simulink model "nucleo_stm32g474_pid_v3_19_05"  (R2025b)
settings: Solver=FixedStepAuto  StartTime=0.0  StopTime=inf  FixedStep=1e-4  RelTol=1e-3  EnableMultiTasking=on
values from neighbouring files (symbols this model uses):
  Ts = single(1e-4)    [smc_mancal.m]
undefined symbols (not defined in the file or in its folder): alpha, dspblkCoreblockFVToolHelper, gcbh
libraries: stm32f4xxblockslib x10, simulink x1
settings Model: STM32="{\"AnalogInput\":[{\"ID\":\"untitled:286\"},{\"ID\":\"untitled:287\"},{\"ID\":\"untitled:288\"},{\"ID\":\"untitled:289\"},{\"ID\":\"nucleo_stm32g474_smc_v1_05_01:311\"},{\"ID\":\"nucleo_stm32g474_smc_v1_05_01:312\"},{\"ID\":\"nucleo_stm32g474_smc_v1_05_01:313\"},{\"ID\":\"nucleo_stm32g474_smc_v1_05_01:314\"},{\"ID\":\"nucleo_stm32g474_smc_v2_06_01:314\"},{\"ID\":\"nucleo_stm32g474_smc_v2_06_01:313\"},{\"ID\":\"nucleo_stm32g474_smc_v2_06_01:312\"},{\"ID\":\"nucleo_stm32g474_smc_v2_06_01:311\"},{\"ID\":\"nucleo_stm32g474_pid_v1_15_01:311\"},{\"ID\":\"nucleo_stm32g474_pid_v1_15_01:312\"},{\"ID\":\"nucleo_stm32g474_pid_v1_15_01:313\"},{\"ID\":\"nucleo_stm32g474_pid_v1_15_01:314\"},{\"ID\":\"nucleo_stm32g474_pid_v1_21_01:311\"},{\"ID\":\"nucleo_stm32g474_pid_v1_21_01:312\"},{\"ID\":\"nucleo_stm32g474_pid_v1_21_01:313\"},{\"ID\":\"nucleo_stm32g474_pid_v1_21_01:314\"},{\"ID\":\"nucleo_stm32g474_pid_v1_29_01:311\"},{\"ID\":\"nucleo_stm32g474_pid_v1_29_01:312\"},{\"ID\":\"nucleo_stm32g474_pid_v1_29_01:313\"},{\"ID\":\"nucleo_stm32g474_pid_v1_29_01:314\"},{\"ID\":\"nucleo_stm32g474_pid_v2_17_03:311\"},{\"ID\":\"nucleo_stm32g474_pid_v2_17_03:312\"},{\"ID\":\"nucleo_stm32g474_pid_v2_17_03:313\"},{\"ID\":\"nucleo_stm32g474_pid_v2_17_03:314\"},{\"ID\":\"nucleo_stm32g474_pid_v3_11_05:311\"},{\"ID\":\"nucleo_stm32g474_pid_v3_11_05:312\"},{\"ID\":\"nucleo_stm32g474_pid_v3_11_05:313\"},{\"ID\":\"nucleo_stm32g474_pid_v3_11_05:314\"},{\"ID\":\"nucleo_stm32g474_pid_v3_19_05:311\"},{\"ID\":\"nucleo_stm32g474_pid_v3_19_05:312\"},{\"ID\":\"nucleo_stm32g474_pid_v3_19_05:313\"},{\"ID\":\"nucleo_stm32g474_pid_v3_19_05:314\"}],\"PWMOutput\":[{\"ID\":\"untitled:236\"},{\"ID\":\"untitled:235\"},{\"ID\":\"untitled:234\"},{\"ID\":\"untitled:233\"},{\"ID\":\"nucleo_stm32g474_smc_v1_05_01:353\"},{\"ID\":\"nucleo_stm32g474_smc_v1_05_01:354\"},{\"ID\":\"nucleo_stm32g474_smc_v1_05_01:355\"},{\"ID\":\"nucleo_stm32g474_smc_v1_05_01:356\"},{\"ID\":\"nucleo_stm32g474_smc_v2_06_01:480\"},{\"ID\":\"nucleo_stm32g474_smc_v2_06_01:481\"},{\"ID\":\"nucleo_stm32g474_smc_v2_06_01:482\"},{\"ID\":\"nucleo_stm32g474_smc_v2_06_01:483\"},{\"ID\":\"nucleo_stm32g474_smc_v2_06_01:488\"},{\"ID\":\"nucleo_stm32g474_pid_v1_15_01:480\"},{\"ID\":\"nucleo_stm32g474_pid_v1_15_01:481\"},{\"ID\":\"nucleo_stm32g474_pid_v1_15_01:482\"},{\"ID\":\"nucleo_stm32g474_pid_v1_15_01:483\"},{\"ID\":\"nucleo_stm32g474_pid_v1_15_01:488\"},{\"ID\":\"nucleo_stm32g474_pid_v1_21_01:480\"},{\"ID\":\"nucleo_stm32g474_pid_v1_21_01:481\"},{\"ID\":\"nucleo_stm32g474_pid_v1_21_01:482\"},{\"ID\":\"nucleo_stm32g474_pid_v1_21_01:483\"},{\"ID\":\"nucleo_stm32g474_pid_v1_21_01:488\"},{\"ID\":\"nucleo_stm32g474_pid_v1_29_01:480\"},{\"ID\":\"nucleo_stm32g474_pid_v1_29_01:481\"},{\"ID\":\"nucleo_stm32g474_pid_v1_29_01:482\"},{\"ID\":\"nucleo_stm32g474_pid_v1_29_01:483\"},{\"ID\":\"nucleo_stm32g474_pid_v1_29_01:488\"},{\"ID\":\"nucleo_stm32g474_pid_v2_17_03:488\"},{\"ID\":\"nucleo_stm32g474_pid_v2_17_03:483\"},{\"ID\":\"nucleo_stm32g474_pid_v2_17_03:482\"},{\"ID\":\"nucleo_stm32g474_pid_v2_17_03:481\"},{\"ID\":\"nucleo_stm32g474_pid_v2_17_03:480\"},{\"ID\":\"nucleo_stm32g474_pid_v3_11_05:480\"},{\"ID\":\"nucleo_stm32g474_pid_v3_11_05:481\"},{\"ID\":\"nucleo_stm32g474_pid_v3_11_05:482\"},{\"ID\":\"nucleo_stm32g474_pid_v3_11_05:483\"},{\"ID\":\"nucleo_stm32g474_pid_v3_11_05:488\"},{\"ID\":\"nucleo_stm32g474_pid_v3_19_05:488\"},{\"ID\":\"nucleo_stm32g474_pid_v3_19_05:483\"},{\"ID\":\"nucleo_stm32g474_pid_v3_19_05:482\"},{\"ID\":\"nucleo_stm32g474_pid_v3_19_05:481\"},{\"ID\":\"nucleo_stm32g474_pid_v3_19_05:480\"}],\"DigitalPortWrite\":{\"ID\":\"nucleo_stm32g474_pid_v3_19_05:665\"}}"  SimulationMode=external  TunableVars=F,lambda,zeta  TunableVarsStorageClass=Auto,Auto,Auto  TunableVarsTypeQualifier=,,  Creator=thaty  LastModifiedBy=thaty
settings OptimizationCC: EnhancedBackFolding=on  PassReuseOutputArgsAs=Individual arguments  ZeroExternalMemoryAtStartup=off  ZeroInternalMemoryAtStartup=off  MaxStackSize=512  OptimizeBlockOrder=speed  DifferentSizesBufferReuse=on  OptimizationCustomize=off  EfficientTunableParamExpr=on
settings DebuggingCC: ParameterTunabilityLossMsg=error
settings HardwareCC: ProdBitPerPointer=32.0  ProdBitPerSizeT=32.0  ProdBitPerPtrDiffT=32.0  ProdLargestAtomicInteger=Long  ProdLargestAtomicFloat=Double  ProdWordSize=32.0  ProdLongLongMode=on  ProdHWDeviceType=ARM Compatible->ARM Cortex-M
settings SFSimCC: MATLABDynamicMemAlloc=off
settings RTWCC: SystemTargetFile=ert.tlc  HardwareBoard=STM32G4xx Based  TemplateMakefile=ert_default_tmf  Toolchain=GNU Tools for ARM Embedded Processors  BuildConfiguration=Faster Runs  Description=Embedded Coder
settings RTWCC: CustomInitializer=|
  | LL_OPAMP_Enable(OPAMP1);
  | LL_OPAMP_Enable(OPAMP2);
  | LL_OPAMP_Enable(OPAMP3);
  | LL_OPAMP_Enable(OPAMP6);
settings CodeAppCC: ForceParamTrailComments=on  IgnoreCustomStorageClasses=off  OperatorAnnotations=on  SimulinkDataObjDesc=on  SFDataObjDesc=on  InsertBlockDesc=on
settings ERTTargetCC: ExtModeTransport=3.0  ExtModeStaticAlloc=on  ExtModeStaticAllocSize=4096.0  ExtModeMexFile=ext_xcp  ExtModeIntrfLevel=Level2 - Open  InlinedParameterPlacement=Hierarchical  TargetLangStandard=C99 (ISO)  CodeReplacementLibrary=ARM Cortex-M

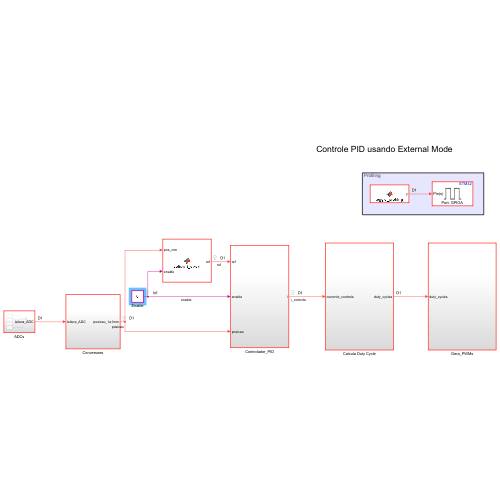
[thumbnail: Simulink's stored preview of the top-level diagram]
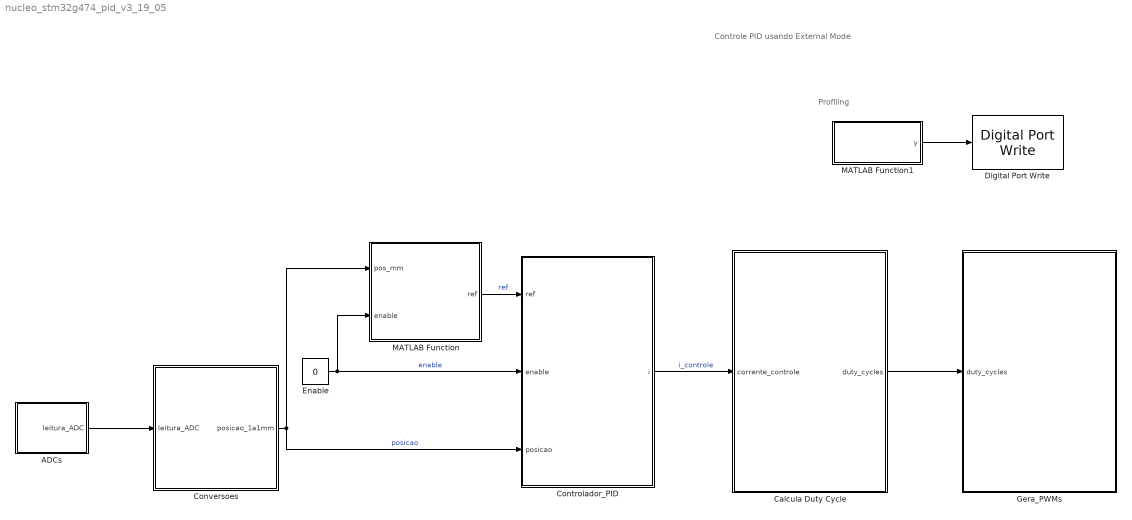
== system nucleo_stm32g474_pid_v3_19_05 ==
  note: Profiling
  note: Controle PID usando External Mode
  ADCs : Subsystem
  Calcula Duty Cycle : Subsystem
  Controlador_PID : Subsystem
  Conversoes : Subsystem
  Digital Port Write : stm32f4xxblockslib/Digital Port Write  PortName=GPIOA  PinNumber=[5]  ReadOperation=off  IOAsArray=on  EnableSimPort=off  hoistedMaskSrc=ECSoC/ECSimCodegen/Digital Port Write
      settings: LibrarySourceBlock=stm32g4xxblockslib/Digital Port Write
  Enable : Constant  Value=0
  Gera_PWMs : Subsystem
  MATLAB Function : MATLAB Function  TreatAsAtomicUnit=on
  MATLAB Function1 : MATLAB Function  TreatAsAtomicUnit=on
  wires:
  ADCs/1(leitura_ADC) -> Conversoes/1(leitura_ADC)
  Conversoes/1(posicao_1a1mm) -> Controlador_PID/3(posicao), MATLAB Function/1(pos_mm)  "posicao"
  Calcula Duty Cycle/1(duty_cycles) -> Gera_PWMs/1(duty_cycles)
  Enable/1 -> MATLAB Function/2(enable), Controlador_PID/2(enable)  "enable"
  MATLAB Function1/1(y) -> Digital Port Write/1
  MATLAB Function/1(ref) -> Controlador_PID/1(ref)  "ref"
  Controlador_PID/1(i) -> Calcula Duty Cycle/1(corrente_controle)  "i_controle"

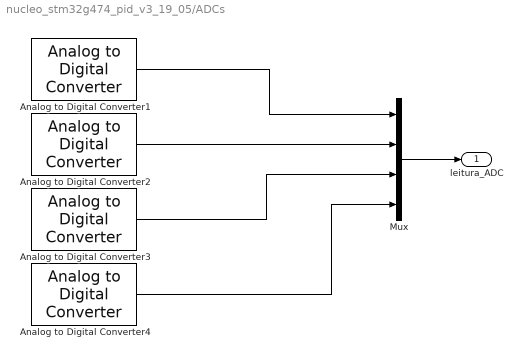
== system nucleo_stm32g474_pid_v3_19_05/ADCs ==
  Analog to Digital Converter1 : stm32f4xxblockslib/Analog to Digital Converter  ADCModule=ADC1  ConversionGroup=Regular  TriggerMode=Read results only  NumberOfConversions=1  EnableBufferConv=off  BufferLength=1  OutputStatus=off  SampleTime=-1  EnableSimPort=off  hoistedMaskSrc=ECSoC/ECSimCodegen/Analog to Digital Converter
  Analog to Digital Converter2 : stm32f4xxblockslib/Analog to Digital Converter  ADCModule=ADC2  ConversionGroup=Regular  TriggerMode=Read results only  NumberOfConversions=1  EnableBufferConv=off  BufferLength=1  OutputStatus=off  SampleTime=-1  EnableSimPort=off  hoistedMaskSrc=ECSoC/ECSimCodegen/Analog to Digital Converter
  Analog to Digital Converter3 : stm32f4xxblockslib/Analog to Digital Converter  ADCModule=ADC3  ConversionGroup=Regular  TriggerMode=Read results only  NumberOfConversions=1  EnableBufferConv=off  BufferLength=1  OutputStatus=off  SampleTime=-1  EnableSimPort=off  hoistedMaskSrc=ECSoC/ECSimCodegen/Analog to Digital Converter
  Analog to Digital Converter4 : stm32f4xxblockslib/Analog to Digital Converter  ADCModule=ADC4  ConversionGroup=Regular  TriggerMode=Read results only  NumberOfConversions=1  EnableBufferConv=off  BufferLength=1  OutputStatus=off  SampleTime=-1  EnableSimPort=off  hoistedMaskSrc=ECSoC/ECSimCodegen/Analog to Digital Converter
  Mux : Mux
  leitura_ADC : Outport
  wires:
  Mux/1 -> leitura_ADC/1
  Analog to Digital Converter1/1 -> Mux/1
  Analog to Digital Converter2/1 -> Mux/2
  Analog to Digital Converter3/1 -> Mux/3
  Analog to Digital Converter4/1 -> Mux/4

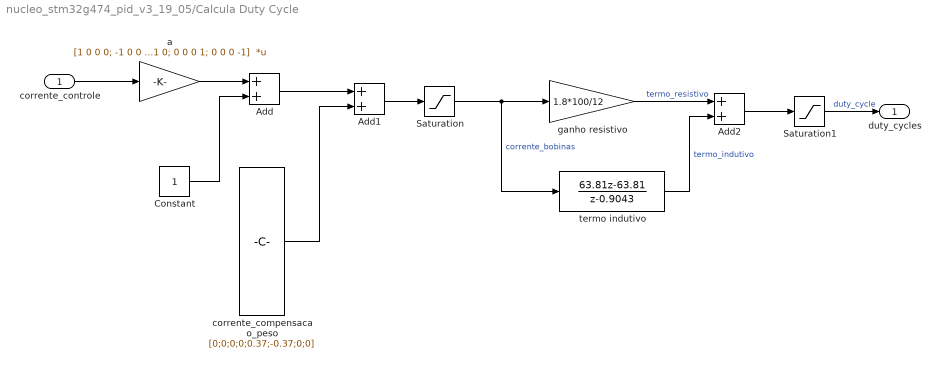
== system nucleo_stm32g474_pid_v3_19_05/Calcula Duty Cycle ==
  corrente_controle : Inport
  Add : Sum  OutDataTypeStr=single  AccumDataTypeStr=single
  Add1 : Sum  OutDataTypeStr=single  AccumDataTypeStr=single
  Add2 : Sum  OutDataTypeStr=single  AccumDataTypeStr=single
  Constant : Constant
  Saturation : Saturate  UpperLimit=3  LowerLimit=0
  Saturation1 : Saturate  UpperLimit=50  LowerLimit=0
  a : Gain  Gain=[1 0 0 0; -1 0 0 0; 0 1 0 0; 0 -1 0 0; 0 0 1 0; 0 0 -1 0; 0 0 0 1; 0 0 0 -1]  Multiplication=Matrix(K*u)  ParamDataTypeStr=single  OutDataTypeStr=single
  corrente_compensacao_peso : Constant  Value=[0;0;0;0;0.37;-0.37;0;0]  VectorParams1D=off  OutDataTypeStr=single
  ganho resistivo : Gain  Gain=1.8*100/12  OutDataTypeStr=single
  termo indutivo : DiscreteTransferFcn  LoadFcn=dspblkCoreblockFVToolHelper(gcbh,'load');  Numerator=[63.81 -63.81]  Denominator=[1 -0.9043]
      settings: CopyFcn=dspblkCoreblockFVToolHelper(gcbh,'copy');  DeleteFcn=dspblkCoreblockFVToolHelper(gcbh,'close');  ModelCloseFcn=dspblkCoreblockFVToolHelper(gcbh,'close');  PreSaveFcn=dspblkCoreblockFVToolHelper(gcbh,'presave');  PostSaveFcn=dspblkCoreblockFVToolHelper(gcbh,'postsave');  CloseFcn=dspblkCoreblockFVToolHelper(gcbh,'close');
  duty_cycles : Outport  VectorParamsAs1DForOutWhenUnconnected=off
  wires:
  Add2/1 -> Saturation1/1
  a/1 -> Add/1
  Add/1 -> Add1/1
  Add1/1 -> Saturation/1
  Saturation/1 -> termo indutivo/1, ganho resistivo/1  "corrente_bobinas"
  corrente_controle/1 -> a/1
  ganho resistivo/1 -> Add2/1  "termo_resistivo"
  termo indutivo/1 -> Add2/2  "termo_indutivo"
  Saturation1/1 -> duty_cycles/1  "duty_cycle"
  Constant/1 -> Add/2
  corrente_compensacao_peso/1 -> Add1/2

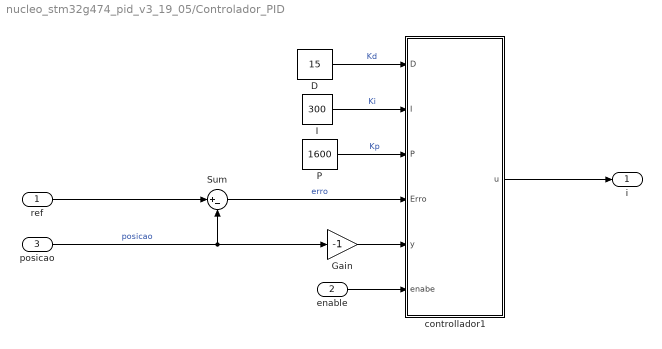
== system nucleo_stm32g474_pid_v3_19_05/Controlador_PID ==
  ref : Inport
  enable : Inport  Port=2
  posicao : Inport  Port=3
  " controllador1" : Subsystem
  D : Constant  Value=15
  Gain : Gain  Gain=-1
  I : Constant  Value=300
  P : Constant  Value=1600
  Sum : Sum  Inputs=|+-  OutDataTypeStr=single  AccumDataTypeStr=single
  i : Outport
  wires:
  ref/1 -> Sum/1
  posicao/1 -> Sum/2, Gain/1  "posicao"
  " controllador1"/1(u) -> i/1
  Sum/1 -> " controllador1"/4(Erro)  "erro"
  Gain/1 -> " controllador1"/5(y)
  P/1 -> " controllador1"/3(P)  "Kp"
  I/1 -> " controllador1"/2(I)  "Ki"
  D/1 -> " controllador1"/1(D)  "Kd"
  enable/1 -> " controllador1"/6(enabe)

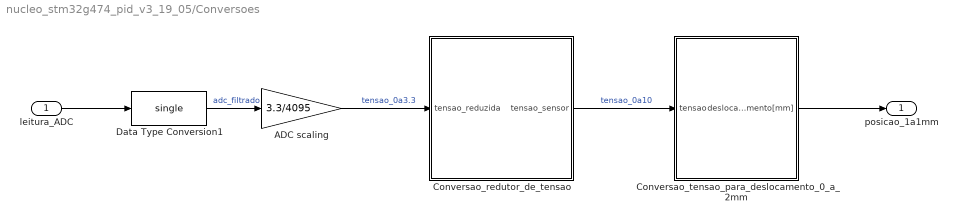
== system nucleo_stm32g474_pid_v3_19_05/Conversoes ==
  leitura_ADC : Inport
  ADC scaling : Gain  Gain=3.3/4095  ParamDataTypeStr=single  OutDataTypeStr=single
  Conversao_redutor_de_tensao : Subsystem
  Conversao_tensao_para_deslocamento_0_a_2mm : Subsystem
  Data Type Conversion1 : DataTypeConversion  OutDataTypeStr=single  SaturateOnIntegerOverflow=off  RndMeth=Floor
  posicao_1a1mm : Outport
  wires:
  Data Type Conversion1/1 -> ADC scaling/1  "adc_filtrado"
  ADC scaling/1 -> Conversao_redutor_de_tensao/1(tensao_reduzida)  "tensao_0a3.3"
  Conversao_redutor_de_tensao/1(tensao_sensor) -> Conversao_tensao_para_deslocamento_0_a_2mm/1(tensao)  "tensao_0a10"
  leitura_ADC/1 -> Data Type Conversion1/1
  Conversao_tensao_para_deslocamento_0_a_2mm/1(deslocamento[mm]) -> posicao_1a1mm/1

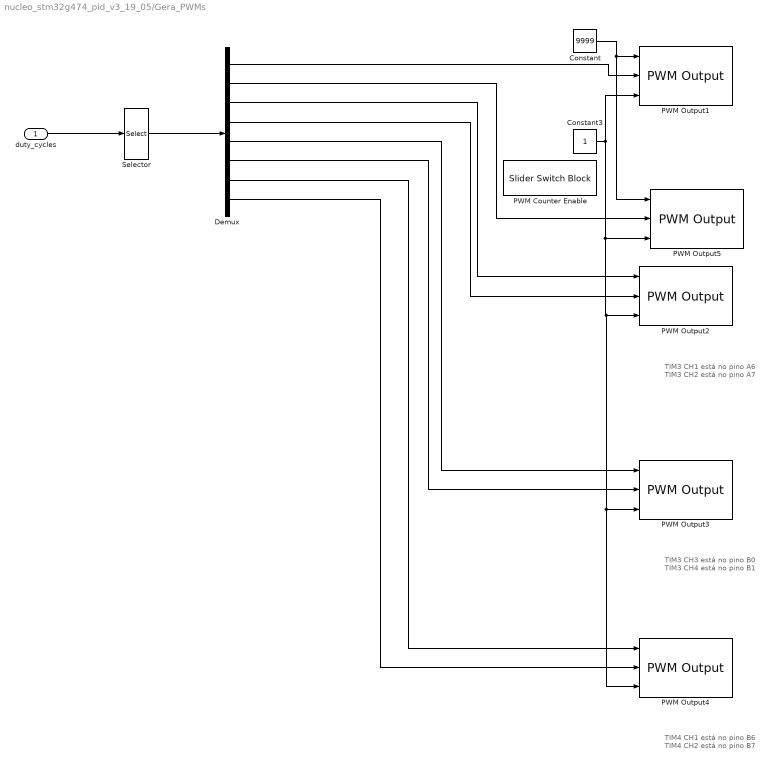
== system nucleo_stm32g474_pid_v3_19_05/Gera_PWMs ==
  note: TIM3 CH1 está no pino A6
      | TIM3 CH2 está no pino A7
  note: TIM3 CH3 está no pino B0
      | TIM3 CH4 está no pino B1
  note: TIM4 CH1 está no pino B6
      | TIM4 CH2 está no pino B7
  duty_cycles : Inport
  Constant : Constant  Value=9999
  Constant3 : Constant
  Demux : Demux  Outputs=8
      settings: DisplayOption=none
  PWM Counter Enable : SliderSwitchBlock  LabelPosition=Hide
  PWM Output1 : stm32f4xxblockslib/PWM Output  ProcessorFamily=STM32F4  TimerModule=TIM8  DutycycleUnits=Percentage  EnableChannel1=on  EnableCaptureCompare1Input=off  EnableCaptureCompare1ComplementaryInput=off  EnableOutputCompare1ModeInput=off  EnableChannel2=off  EnableCaptureCompare2Input=off  EnableCaptureCompare2ComplementaryInput=off  EnableOutputCompare2ModeInput=off  EnableChannel3=off  EnableCaptureCompare3Input=off  EnableCaptureCompare3ComplementaryInput=off  EnableOutputCompare3ModeInput=off  EnableChannel4=off  EnableCaptureCompare4Input=off  EnableCaptureCompare4ComplementaryInput=off  EnableOutputCompare4ModeInput=off  EnableChannel5=off  EnableCaptureCompare5Input=off  EnableOutputCompare5ModeInput=off  EnableChannel6=off  EnableCaptureCompare6Input=off  EnableOutputCompare6ModeInput=off  EnableCounterInput=on  EnableMainOutputInput=off  EnableFrequencyInput=on  SetRCAfterCE=off  OutputDirection=off  OutputMainOutputEnableStatus=off  SampleTime=0.1  EnableSimPort=off  EnableUpdateEvent=off  EnableCaptureCompare1Event=off  EnableCaptureCompare2Event=off  EnableCaptureCompare3Event=off  EnableCaptureCompare4Event=off  EnableTriggerEvent=off  EnableBreakEvent=off  EnableBreakEvent2=off  hoistedMaskSrc=ECSoC/ECSimCodegen/PWM Output
  PWM Output2 : stm32f4xxblockslib/PWM Output  ProcessorFamily=STM32F4  TimerModule=TIM3  DutycycleUnits=Percentage  EnableChannel1=on  EnableCaptureCompare1Input=off  EnableCaptureCompare1ComplementaryInput=off  EnableOutputCompare1ModeInput=off  EnableChannel2=on  EnableCaptureCompare2Input=off  EnableCaptureCompare2ComplementaryInput=off  EnableOutputCompare2ModeInput=off  EnableChannel3=off  EnableCaptureCompare3Input=off  EnableCaptureCompare3ComplementaryInput=off  EnableOutputCompare3ModeInput=off  EnableChannel4=off  EnableCaptureCompare4Input=off  EnableCaptureCompare4ComplementaryInput=off  EnableOutputCompare4ModeInput=off  EnableChannel5=off  EnableCaptureCompare5Input=off  EnableOutputCompare5ModeInput=off  EnableChannel6=off  EnableCaptureCompare6Input=off  EnableOutputCompare6ModeInput=off  EnableCounterInput=on  EnableMainOutputInput=off  EnableFrequencyInput=off  SetRCAfterCE=off  OutputDirection=off  OutputMainOutputEnableStatus=off  SampleTime=0.1  EnableSimPort=off  EnableUpdateEvent=off  EnableCaptureCompare1Event=off  EnableCaptureCompare2Event=off  EnableCaptureCompare3Event=off  EnableCaptureCompare4Event=off  EnableTriggerEvent=off  EnableBreakEvent=off  EnableBreakEvent2=off  hoistedMaskSrc=ECSoC/ECSimCodegen/PWM Output
  PWM Output3 : stm32f4xxblockslib/PWM Output  ProcessorFamily=STM32F4  TimerModule=TIM3  DutycycleUnits=Percentage  EnableChannel1=off  EnableCaptureCompare1Input=off  EnableCaptureCompare1ComplementaryInput=off  EnableOutputCompare1ModeInput=off  EnableChannel2=off  EnableCaptureCompare2Input=off  EnableCaptureCompare2ComplementaryInput=off  EnableOutputCompare2ModeInput=off  EnableChannel3=on  EnableCaptureCompare3Input=off  EnableCaptureCompare3ComplementaryInput=off  EnableOutputCompare3ModeInput=off  EnableChannel4=on  EnableCaptureCompare4Input=off  EnableCaptureCompare4ComplementaryInput=off  EnableOutputCompare4ModeInput=off  EnableChannel5=off  EnableCaptureCompare5Input=off  EnableOutputCompare5ModeInput=off  EnableChannel6=off  EnableCaptureCompare6Input=off  EnableOutputCompare6ModeInput=off  EnableCounterInput=on  EnableMainOutputInput=off  EnableFrequencyInput=off  SetRCAfterCE=off  OutputDirection=off  OutputMainOutputEnableStatus=off  SampleTime=0.1  EnableSimPort=off  EnableUpdateEvent=off  EnableCaptureCompare1Event=off  EnableCaptureCompare2Event=off  EnableCaptureCompare3Event=off  EnableCaptureCompare4Event=off  EnableTriggerEvent=off  EnableBreakEvent=off  EnableBreakEvent2=off  hoistedMaskSrc=ECSoC/ECSimCodegen/PWM Output
  PWM Output4 : stm32f4xxblockslib/PWM Output  ProcessorFamily=STM32F4  TimerModule=TIM4  DutycycleUnits=Percentage  EnableChannel1=on  EnableCaptureCompare1Input=off  EnableCaptureCompare1ComplementaryInput=off  EnableOutputCompare1ModeInput=off  EnableChannel2=on  EnableCaptureCompare2Input=off  EnableCaptureCompare2ComplementaryInput=off  EnableOutputCompare2ModeInput=off  EnableChannel3=off  EnableCaptureCompare3Input=off  EnableCaptureCompare3ComplementaryInput=off  EnableOutputCompare3ModeInput=off  EnableChannel4=off  EnableCaptureCompare4Input=off  EnableCaptureCompare4ComplementaryInput=off  EnableOutputCompare4ModeInput=off  EnableChannel5=off  EnableCaptureCompare5Input=off  EnableOutputCompare5ModeInput=off  EnableChannel6=off  EnableCaptureCompare6Input=off  EnableOutputCompare6ModeInput=off  EnableCounterInput=on  EnableMainOutputInput=off  EnableFrequencyInput=off  SetRCAfterCE=off  OutputDirection=off  OutputMainOutputEnableStatus=off  SampleTime=0.1  EnableSimPort=off  EnableUpdateEvent=off  EnableCaptureCompare1Event=off  EnableCaptureCompare2Event=off  EnableCaptureCompare3Event=off  EnableCaptureCompare4Event=off  EnableTriggerEvent=off  EnableBreakEvent=off  EnableBreakEvent2=off  hoistedMaskSrc=ECSoC/ECSimCodegen/PWM Output
  PWM Output5 : stm32f4xxblockslib/PWM Output  ProcessorFamily=STM32F4  TimerModule=TIM4  DutycycleUnits=Percentage  EnableChannel1=off  EnableCaptureCompare1Input=off  EnableCaptureCompare1ComplementaryInput=off  EnableOutputCompare1ModeInput=off  EnableChannel2=off  EnableCaptureCompare2Input=off  EnableCaptureCompare2ComplementaryInput=off  EnableOutputCompare2ModeInput=off  EnableChannel3=off  EnableCaptureCompare3Input=off  EnableCaptureCompare3ComplementaryInput=off  EnableOutputCompare3ModeInput=off  EnableChannel4=on  EnableCaptureCompare4Input=off  EnableCaptureCompare4ComplementaryInput=off  EnableOutputCompare4ModeInput=off  EnableChannel5=off  EnableCaptureCompare5Input=off  EnableOutputCompare5ModeInput=off  EnableChannel6=off  EnableCaptureCompare6Input=off  EnableOutputCompare6ModeInput=off  EnableCounterInput=on  EnableMainOutputInput=off  EnableFrequencyInput=on  SetRCAfterCE=off  OutputDirection=off  OutputMainOutputEnableStatus=off  SampleTime=0.1  EnableSimPort=off  EnableUpdateEvent=off  EnableCaptureCompare1Event=off  EnableCaptureCompare2Event=off  EnableCaptureCompare3Event=off  EnableCaptureCompare4Event=off  EnableTriggerEvent=off  EnableBreakEvent=off  EnableBreakEvent2=off  hoistedMaskSrc=ECSoC/ECSimCodegen/PWM Output
  Selector : Selector  InputPortWidth=8  IndexOptions=Index vector (dialog)  Indices=[1 2 3 4 6 5 7 8]  OutputSizes=1
  wires:
  Constant3/1 -> PWM Output5/3, PWM Output4/3, PWM Output3/3, PWM Output2/3, PWM Output1/3
  Demux/1 -> PWM Output1/2
  Demux/5 -> PWM Output3/1
  Demux/6 -> PWM Output3/2
  Constant/1 -> PWM Output5/1, PWM Output1/1
  Demux/3 -> PWM Output2/1
  Demux/4 -> PWM Output2/2
  Demux/7 -> PWM Output4/1
  Demux/8 -> PWM Output4/2
  Demux/2 -> PWM Output5/2
  duty_cycles/1 -> Selector/1
  Selector/1 -> Demux/1

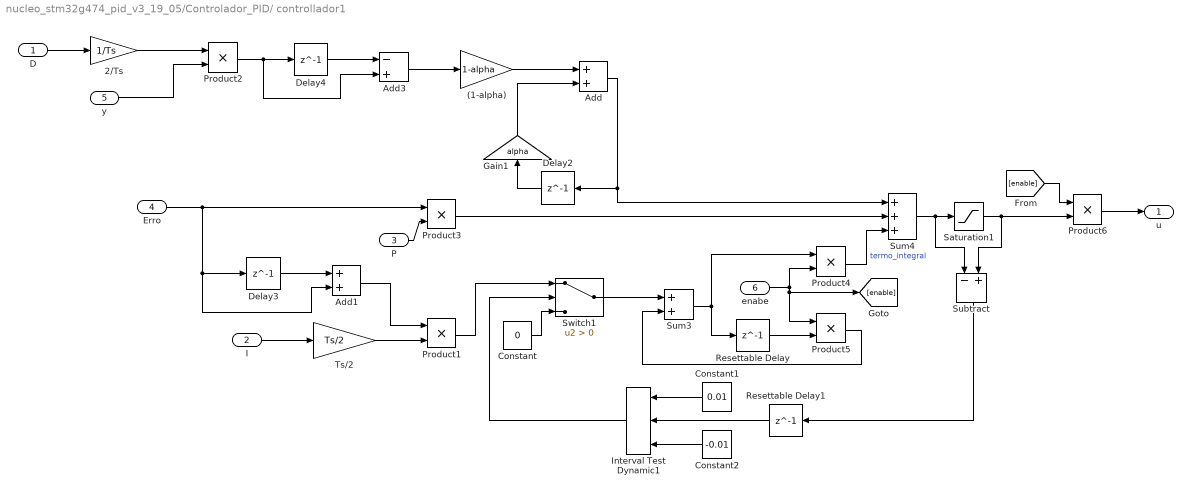
== system nucleo_stm32g474_pid_v3_19_05/Controlador_PID/ controllador1 ==
  D : Inport
  I : Inport  Port=2
  P : Inport  Port=3
  Erro : Inport  Port=4
  y : Inport  Port=5
  enabe : Inport  Port=6
  (1-alpha) : Gain  Gain=1-alpha
  2/Ts : Gain  Gain=1/Ts  ParamDataTypeStr=single  OutDataTypeStr=single
  Add : Sum
  Add1 : Sum
  Add3 : Sum  Inputs=-+
  Constant : Constant  Value=0  OutDataTypeStr=single
  Constant1 : Constant  Value=0.01  OutDataTypeStr=single
  Constant2 : Constant  Value=-0.01  OutDataTypeStr=single
  Delay2 : Delay  DelayLength=1
  Delay3 : Delay  DelayLength=1
  Delay4 : Delay  DelayLength=1
  Gain1 : Gain  Gain=alpha
  Interval Test Dynamic1 : simulink/Logic and Bit Operations/Interval Test Dynamic  IntervalClosedRight=on  IntervalClosedLeft=on  OutDataTypeStr=boolean
  Product{1..6} (6 alike) : Product  OutDataTypeStr=single
  Resettable Delay : Delay  DelayLength=1
  Resettable Delay1 : Delay  DelayLength=1
  Saturation1 : Saturate  UpperLimit=2  LowerLimit=-2
  Subtract : Sum  Inputs=-+  OutDataTypeStr=single  AccumDataTypeStr=single
  Sum3 : Sum  OutDataTypeStr=single  AccumDataTypeStr=single
  Sum4 : Sum  Inputs=+++  OutDataTypeStr=single  AccumDataTypeStr=single
  Switch1 : Switch  Criteria=u2 > Threshold  OutDataTypeStr=single  SaturateOnIntegerOverflow=off  InputSameDT=off
  Ts/2 : Gain  Gain=Ts/2  ParamDataTypeStr=single  OutDataTypeStr=single
  u : Outport  VectorParamsAs1DForOutWhenUnconnected=off
  wires:
  Constant/1 -> Switch1/3
  Delay2/1 -> Gain1/1
  Constant2/1 -> Interval Test Dynamic1/3
  Sum4/1 -> Saturation1/1, Subtract/1
  I/1 -> Ts/2/1
  P/1 -> Product3/2
  (1-alpha)/1 -> Add/1
  2/Ts/1 -> Product2/1
  Add1/1 -> Product1/1
  D/1 -> 2/Ts/1
  Constant1/1 -> Interval Test Dynamic1/1
  Ts/2/1 -> Product1/2
  Subtract/1 -> Resettable Delay1/1
  Sum3/1 -> Product4/1, Resettable Delay/1
  Erro/1 -> Product3/1, Add1/2, Delay3/1
  Gain1/1 -> Add/2
  Delay3/1 -> Add1/1
  Add/1 -> Sum4/1, Delay2/1
  Delay4/1 -> Add3/1
  Product1/1 -> Switch1/1
  Product3/1 -> Sum4/2
  Switch1/1 -> Sum3/1
  Product2/1 -> Add3/2, Delay4/1
  Resettable Delay1/1 -> Interval Test Dynamic1/2
  Interval Test Dynamic1/1 -> Switch1/2
  Saturation1/1 -> Subtract/2, Product6/2
  Add3/1 -> (1-alpha)/1
  y/1 -> Product2/2
  Product4/1 -> Sum4/3  "termo_integral"
  Product5/1 -> Sum3/2
  enabe/1 -> [enable], Product5/1, Product4/2
  Resettable Delay/1 -> Product5/2
  [enable] -> Product6/1
  Product6/1 -> u/1

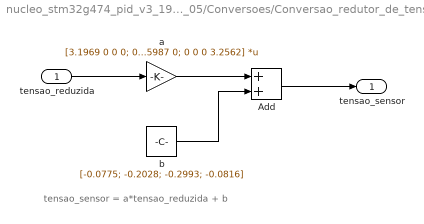
== system nucleo_stm32g474_pid_v3_19_05/Conversoes/Conversao_redutor_de_tensao ==
  note: tensao_sensor = a*tensao_reduzida + b
  tensao_reduzida : Inport
  Add : Sum  OutDataTypeStr=single  AccumDataTypeStr=single
  a : Gain  Gain=[3.1969 0 0 0; 0 3.415 0 0; 0 0 3.5987 0; 0 0 0 3.2562]  Multiplication=Matrix(K*u)  ParamDataTypeStr=single  OutDataTypeStr=single
  b : Constant  Value=[-0.0775; -0.2028; -0.2993; -0.0816]  OutDataTypeStr=single
  tensao_sensor : Outport
  wires:
  tensao_reduzida/1 -> a/1
  a/1 -> Add/1
  b/1 -> Add/2
  Add/1 -> tensao_sensor/1

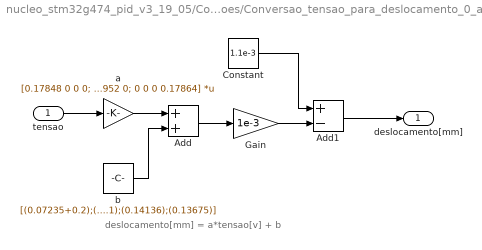
== system nucleo_stm32g474_pid_v3_19_05/Conversoes/Conversao_tensao_para_deslocamento_0_a_2mm ==
  note: deslocamento[mm] = a*tensao[v] + b
  tensao : Inport
  Add : Sum  OutDataTypeStr=single  AccumDataTypeStr=single
  Add1 : Sum  Inputs=+-
  Constant : Constant  Value=1.1e-3
  Gain : Gain  Gain=1e-3
  a : Gain  Gain=[0.17848 0 0 0; 0 0.17816 0 0; 0 0 0.17952 0; 0 0 0 0.17864]  Multiplication=Matrix(K*u)  ParamDataTypeStr=single  OutDataTypeStr=single
  b : Constant  Value=[(0.07235+0.2);(0.12782+0.1);(0.14136);(0.13675)]  OutDataTypeStr=single
  deslocamento[mm] : Outport
  wires:
  tensao/1 -> a/1
  a/1 -> Add/1
  b/1 -> Add/2
  Add/1 -> Gain/1
  Add1/1 -> deslocamento[mm]/1
  Constant/1 -> Add1/1
  Gain/1 -> Add1/2

== matlab function nucleo_stm32g474_pid_v3_19_05/MATLAB Function ==
  data: pos_mm input; ref output; enable input
function ref = softstart_eixoY(pos_mm, enable)
%#codegen
% ENTRADAS:
%   pos_mm : posicao dos 4 sensores em mm, ordem [Ya, Xa, Yb, Xb]
%   enable : 0 antes da partida, 1 dispara a levitacao
% SAIDA:
%   ref    : setpoint dos 4 eixos em mm (-> Controlador_PID/ref)
%
% Ordem dos sinais (CONFIRMADA): [Ya, Xa, Yb, Xb]
%   indice 1 = Ya (vertical, Mancal A)   -> recebe rampa
%   indice 2 = Xa (horizontal, Mancal A) -> segue posicao (passivo)
%   indice 3 = Yb (vertical, Mancal B)   -> recebe rampa
%   indice 4 = Xb (horizontal, Mancal B) -> segue posicao (passivo)

% ----- AJUSTE AO SEU PROJETO -----
    IDX_VERT = [1 2 3 4];            % indices dos eixos verticais (Ya, Yb)
    Ts       = single(1e-4);    % periodo de controle [s] (10 kHz)
    T_RAMPA  = single(0.1);       % duracao da rampa ate o centro [s]
% ---------------------------------

    persistent sp_ini t_acc started
    if isempty(started)
        started = false;
        sp_ini  = single([0;0;0;0]);
        t_acc   = single(0);
    end

    p = single(pos_mm(:));

    % Base: TODOS os eixos seguem a posicao medida
    % (erro ~ 0, corrente ~ 0 nos eixos nao controlados)
    ref = p;

    if enable < 0.5
        sp_ini  = p;
        t_acc   = single(0);
        started = false;
        ref     = single(ref);
        return;
    end

    % enable subiu para 1: congela o ponto de partida
    if ~started
        sp_ini  = p;
        t_acc   = single(0);
        started = true;
    end

    % Rampa nos DOIS eixos verticais (Ya e Yb): de sp_ini -> 0 (centro)
    if t_acc < T_RAMPA
        frac = t_acc / T_RAMPA;             % 0 -> 1
        for k = 1:numel(IDX_VERT)
            idx = IDX_VERT(k);
            ref(idx) = sp_ini(idx) * (single(1) - frac);
        end
        t_acc = t_acc + Ts;
    else
        for k = 1:numel(IDX_VERT)
            ref(IDX_VERT(k)) = single(0);  % ambos no centro
        end
    end

    % Eixos horizontais (2=Xa, 4=Xb) permanecem = posicao medida
    ref = single(ref);
end

== matlab function nucleo_stm32g474_pid_v3_19_05/MATLAB Function1 ==
  data: y output
function y = toggle_profiling()
%#codegen
% Inverte o estado a cada execucao do step.
% Saida y (uint8): 0 ou 1, vai direto para o pino GPIO.

    persistent s
    if isempty(s)
        s = false;
    end
    s = ~s;
    y = uint8(s);
end
